simulink model "ex10"  (R2020a)
settings: Solver=ode45  StartTime=0.0  StopTime=10  RelTol=1e-3
settings Model: Creator=반달  LastModifiedBy=반달
settings DataIOCC: ReturnWorkspaceOutputs=off

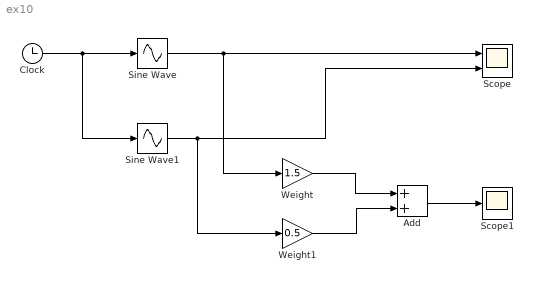
== system ex10 ==
  Add : Sum
  Clock : Clock
  Scope : Scope  NumInputPorts=2
  Scope1 : Scope
  Sine Wave : Sin  TimeSource=Use external signal  Frequency=2*pi*1/4  SampleTime=0
  Sine Wave1 : Sin  TimeSource=Use external signal  Frequency=2*pi*1/6  SampleTime=0
  Weight : Gain  Gain=1.5
  Weight1 : Gain  Gain=0.5
  wires:
  Clock/1 -> Sine Wave1/1, Sine Wave/1
  Sine Wave/1 -> Weight/1, Scope/1
  Sine Wave1/1 -> Weight1/1, Scope/2
  Weight/1 -> Add/1
  Weight1/1 -> Add/2
  Add/1 -> Scope1/1
